simulink model "Loadcell_Reader"  (R2024b)
settings: Solver=FixedStepAuto  StartTime=0.0  StopTime=10  FixedStep=0.01  RelTol=1e-3  EnableMultiTasking=on
libraries: stm32f4xxblockslib x1
settings Model: STM32="{\"AnalogInput\":[{\"ID\":\"BasicKit:1\"},{\"ID\":\"Potentiometer_Reader:1\"},{\"ID\":\"Loadcell_Reader:1\"}],\"DigitalPortWrite\":{\"ID\":\"BasicKit:4\"},\"DigitalPortRead\":[{\"ID\":\"BasicKit:5\"},{\"ID\":\"BasicKit:7\"}]}"  Creator=pboon  LastModifiedBy=pboon
settings OptimizationCC: DefaultParameterBehavior=Inlined  EnhancedBackFolding=on  PassReuseOutputArgsAs=Individual arguments  ZeroExternalMemoryAtStartup=off  ZeroInternalMemoryAtStartup=off  MaxStackSize=512  OptimizeBlockOrder=speed  DifferentSizesBufferReuse=on  OptimizationCustomize=off  EfficientTunableParamExpr=on
settings DebuggingCC: ParameterTunabilityLossMsg=error
settings HardwareCC: ProdBitPerPointer=32  ProdBitPerSizeT=32  ProdBitPerPtrDiffT=32  ProdLargestAtomicInteger=Long  ProdLargestAtomicFloat=Double  ProdWordSize=32  ProdLongLongMode=on  ProdHWDeviceType=ARM Compatible->ARM Cortex-M
settings SFSimCC: MATLABDynamicMemAlloc=off
settings RTWCC: Description=Embedded Coder  SystemTargetFile=ert.tlc  HardwareBoard=STM32G4xx Based  TemplateMakefile=ert_default_tmf  Toolchain=GNU Tools for ARM Embedded Processors
settings CodeAppCC: ForceParamTrailComments=on  IgnoreCustomStorageClasses=off  OperatorAnnotations=on  SimulinkDataObjDesc=on  SFDataObjDesc=on  InsertBlockDesc=on
settings ERTTargetCC: TargetLangStandard=C99 (ISO)  CodeReplacementLibrary=ARM Cortex-M  ExtModeTransport=3  ExtModeStaticAlloc=on  ExtModeStaticAllocSize=2048  ExtModeMexFile=ext_xcp  ExtModeIntrfLevel=Level2 - Open

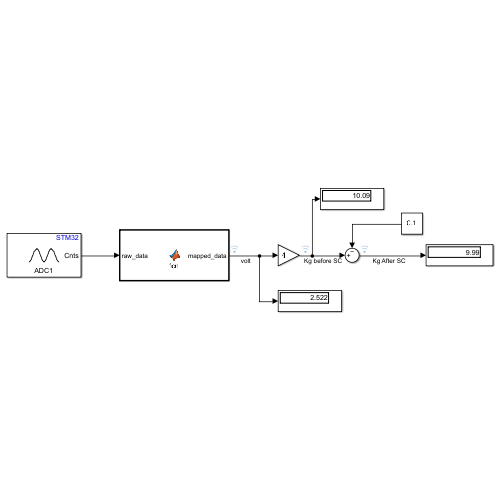
[thumbnail: Simulink's stored preview of the top-level diagram]
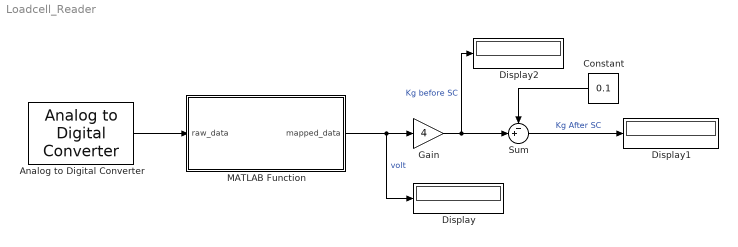
== system Loadcell_Reader ==
  Analog to Digital Converter : stm32f4xxblockslib/Analog to Digital Converter  ADCModule=ADC1  ConversionGroup=Regular  TriggerMode=Trigger and read  NumberOfConversions=1  EnableBufferConv=off  BufferLength=1  OutputStatus=off  SampleTime=-1  EnableSimPort=off  hoistedMaskSrc=ECSoC/ECSimCodegen/Analog to Digital Converter
  Constant : Constant  Value=0.1
  Display : Display
  Display1 : Display
      settings: Format=bank
  Display2 : Display
  Gain : Gain  Gain=4
  MATLAB Function : MATLAB Function  TreatAsAtomicUnit=on
  Sum : Sum  Inputs=-+|
  wires:
  MATLAB Function/1(mapped_data) -> Display/1, Gain/1  "volt"
  Analog to Digital Converter/1 -> MATLAB Function/1(raw_data)
  Gain/1 -> Display2/1, Sum/2  "Kg before SC"
  Constant/1 -> Sum/1
  Sum/1 -> Display1/1  "Kg After SC"

== matlab function Loadcell_Reader/MATLAB Function ==
  data: raw_data input; mapped_data output
function mapped_data = fcn(raw_data)

in_min = 0.0;
out_min = 0.0;
in_max = 4095.0;
out_max = 3.3;

mapped_data =  (double(raw_data) - in_min) * (out_max - out_min) / (in_max - in_min) + out_min;
